simulink model "Elevator_lift"  (R2024b)
settings: Solver=VariableStepAuto  StartTime=0.0  StopTime=inf  RelTol=1e-3
settings Model: PacingRate=0.089000  Creator=HP  LastModifiedBy=HP

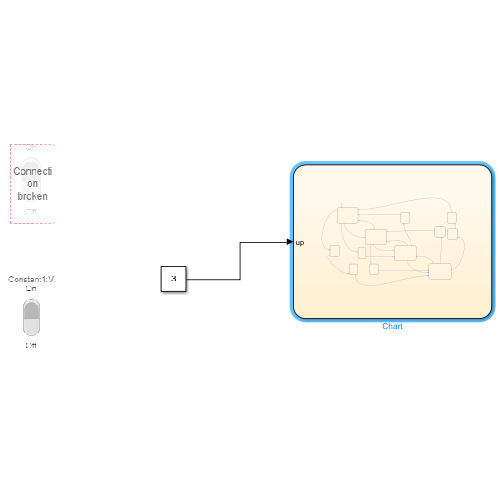
[thumbnail: Simulink's stored preview of the top-level diagram]
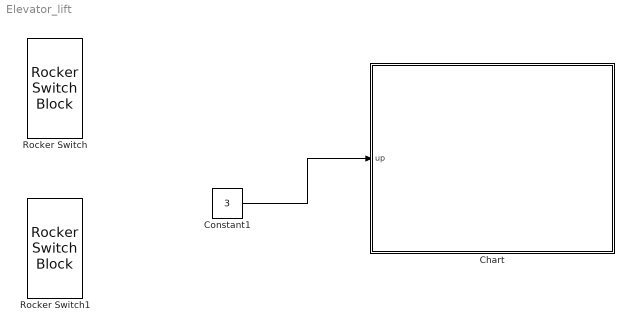
== system Elevator_lift ==
  Chart : Stateflow chart  TreatAsAtomicUnit=on
  Constant1 : Constant  Value=3
  Rocker Switch : RockerSwitchBlock
      settings: Values={{'Off', 'On'}, [0 1]}
  Rocker Switch1 : RockerSwitchBlock
      settings: Values={{'Off', 'On'}, [0 1]}
  wires:
  Constant1/1 -> Chart/1(up)

== stateflow chart Elevator_lift/Chart ==
  state Ground
    entry:
    door=1;
    exit:
    door=0;
  state first3
    entry:
    door=0;
  state first2
    entry:
    door=0;
  state second3
    entry:
    door=0;
  state second2
    entry:
    door=0;
  state first
    entry:
    door=1;
    exit:
    door=0;
  state first1
    entry:
    door=0;
  state second
    entry:
    door=1;
    exit:
    door=0;
  state first4
    entry:
    door=0;
  state third
    entry:
    door=1;
    exit:
    door=0;
  state second1
    entry:
    door=0;
  state second4
    entry:
    door=0;
  first2 -> Ground
  (default) -> Ground
  Ground -> first1 [order 3] : [up==3]
  first3 -> Ground
  first -> Ground [order 2] : [up==0]
  Ground -> first4 [order 2] : [up==2]
  Ground -> first [order 1] : [up==1]
  second -> first3 [order 3] : [up==0]
  second2 -> first2
  second3 -> first
  third -> second2 [order 1] : [up==0]
  third -> second3 [order 3] : [up==1]
  second -> first [order 2] : [up==1]
  first -> second4 [order 3] : [up==3]
  first -> second [order 1] : [up==2]
  first1 -> second1
  third -> second [order 2] : [up==2]
  first4 -> second
  second -> third [order 1] : [up==3]
  second4 -> third
  second1 -> third
  data: up input; door local
